simulink model "studio3_partb"  (R2020a)
settings: Solver=ode45  StartTime=-1  StopTime=20  FixedStep=0.2  MaxStep=0.05  RelTol=1e-8  AbsTol=1e-8  EnableMultiTasking=on
settings Model: ExtModeTrigMode=oneshot  ExtModeArmWhenConnect=off  Creator=LEVIENKL  LastModifiedBy=Vy Possible
settings SolverCC: AutoScaleAbsTol=off
settings DataIOCC: SaveFormat=Array  SignalLoggingSaveFormat=ModelDataLogs  SaveOutput=off  SaveTime=off  ReturnWorkspaceOutputs=off  SignalLoggingName=sigsOut
settings OptimizationCC: BlockReduction=off  BooleanDataType=off  ExpressionDepthLimit=2147483647  InitFltsAndDblsToZero=on  LifeSpan=inf
settings DebuggingCC: SaveWithParameterizedLinksMsg=none  UnderspecifiedInitializationDetection=Classic  MergeDetectMultiDrivingBlocksExec=none  SignalResolutionControl=TryResolveAllWithWarning  MultiTaskDSMMsg=warning  MultiTaskCondExecSysMsg=none  FcnCallInpInsideContextMsg=warning  AllowSymbolicDim=off  StateNameClashWarn=warning  SFUnexpectedBacktrackingDiag=warning  SFNoUnconditionalDefaultTransitionDiag=warning  SFExecutionAtInitializationDiag=none  ArithmeticOperatorsInVariantConditions=warning
settings HardwareCC: ProdBitPerPointer=32  ProdBitPerSizeT=32  ProdBitPerPtrDiffT=32  ProdLargestAtomicFloat=None  ProdIntDivRoundTo=Undefined  ProdEndianess=Unspecified  ProdWordSize=32  ProdHWDeviceType=32-bit Generic  TargetUnknown=on
settings ModelReferenceCC: PropagateSignalLabelsOutOfModel=off
settings SFSimCC: SimUseLocalCustomCode=off  CustomCodeUndefinedFunction=UseInterfaceOnly
settings RTWCC: RTWUseLocalCustomCode=off
settings CodeAppCC: StateflowObjectComments=on
settings GRTTargetCC: TargetFcnLib=ansi_tfl_tmw.mat  TargetLangStandard=C89/C90 (ANSI)  CombineOutputUpdateFcns=off  GRTInterface=on
settings ConfigComp: CovMetricSettings=dw  CovHtmlReporting=on  CovSaveCumulativeToWorkspaceVar=on  CovSaveSingleToWorkspaceVar=on  CovExternalEMLEnable=off  CovSFcnEnable=off

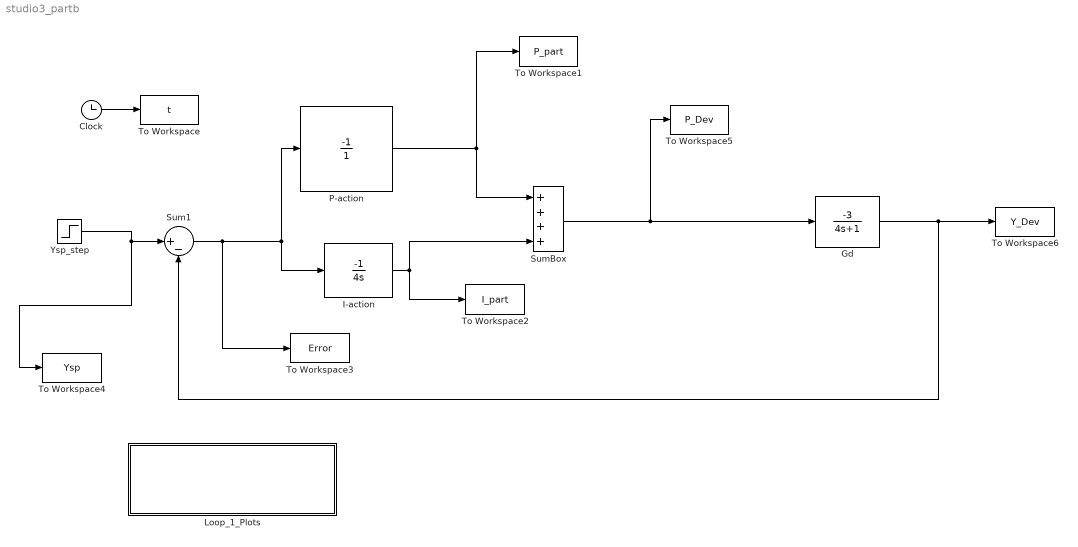
== system studio3_partb ==
  Clock : Clock
  Gd : TransferFcn  Numerator=[-3]  Denominator=[4 1]
  "I-action " : TransferFcn  Numerator=[-1]  Denominator=[4,0]
  Loop_1_Plots : Subsystem  mask(Y,U,E Plots - Loop 1){}
      settings: OpenFcn=YPEplots
      mask Help: This block loop #1 Y,U,Error in 3x1 Figure Window.
      mask Display: disp('After Loop 1 Simulation:\n Double Click for Y, P, Error Plots\n (uses YPEplots.p)')
  "P-action " : TransferFcn  Numerator=[-1]  Denominator=[0 1]
  Sum1 : Sum  Inputs=|+-  InputSameDT=on  SaturateOnIntegerOverflow=on  OutDataTypeStr=Inherit: Same as first input
  SumBox : Sum  Inputs=++++
  To Workspace : ToWorkspace  VariableName=t  SampleTime=-1
  To Workspace1 : ToWorkspace  VariableName=P_part  SampleTime=-1
  To Workspace2 : ToWorkspace  VariableName=I_part  SampleTime=-1
  To Workspace3 : ToWorkspace  VariableName=Error  SampleTime=-1
  To Workspace4 : ToWorkspace  VariableName=Ysp  SampleTime=-1
  To Workspace5 : ToWorkspace  VariableName=P_Dev  SampleTime=-1
  To Workspace6 : ToWorkspace  VariableName=Y_Dev  SampleTime=-1
  Ysp_step : Step  Time=0  After=12  SampleTime=0
      settings: AttributesFormatString=%<Before> to %<After>\nat %<Time>
  wires:
  Clock/1 -> To Workspace/1
  Gd/1 -> Sum1/2, To Workspace6/1
  Ysp_step/1 -> To Workspace4/1, Sum1/1
  Sum1/1 -> To Workspace3/1, "P-action "/1, "I-action "/1
  "P-action "/1 -> To Workspace1/1, SumBox/1
  "I-action "/1 -> To Workspace2/1, SumBox/4
  SumBox/1 -> To Workspace5/1, Gd/1

== system studio3_partb/Loop_1_Plots ==
